simulink model "EL5101"  (Simulink 9.2)
settings: Solver=FixedStepDiscrete  StartTime=0.0  StopTime=inf  FixedStep=param.t_sample  RelTol=1e-3
undefined symbols (not defined in the file or in its folder): Angle_deg
libraries: simulink_extras x1, etherlab_lib x1
settings Model: Creator=schappler  LastModifiedBy=pkr_devpc  SimulationMode=external  ExtModeTrigDuration=10000  ExtModeArchiveMode=auto  ExtModeArchiveFileName=measurement_data  ExtModeArchiveDirName=/home/pkr_devpc/Schreibtisch/Git/3rrr_pkm/Versuchsstand/result  ExtModeLogAll=off
settings SolverCC: MinimalZcImpactIntegration=on
settings DataIOCC: LimitDataPoints=off  SaveFormat=Dataset  SignalLoggingSaveFormat=Dataset  SaveOutput=off  SignalLogging=off  SaveTime=off
settings OptimizationCC: BufferReuse=off  GlobalBufferReuse=off  ExpressionFolding=off  LocalBlockOutputs=off  LifeSpan=auto  OptimizeDataStoreBuffers=off  BusAssignmentInplaceUpdate=off
settings DebuggingCC: ReadBeforeWriteMsg=DisableAll  WriteAfterWriteMsg=DisableAll  WriteAfterReadMsg=DisableAll  UnderspecifiedInitializationDetection=Simplified  MergeDetectMultiDrivingBlocksExec=error  MultiTaskDSMMsg=none  FcnCallInpInsideContextMsg=error  StateNameClashWarn=none  SFUnexpectedBacktrackingDiag=error  SFNoUnconditionalDefaultTransitionDiag=error  SFExecutionAtInitializationDiag=warning
settings HardwareCC: ProdBitPerPointer=64  ProdBitPerSizeT=64  ProdBitPerPtrDiffT=64  ProdLargestAtomicFloat=Float  ProdIntDivRoundTo=Zero  ProdEndianess=LittleEndian  ProdWordSize=64  ProdHWDeviceType=Intel->x86-64 (Windows64)
settings ModelReferenceCC: UpdateModelReferenceTargets=IfOutOfDate  PropagateSignalLabelsOutOfModel=on
settings SFSimCC: SFSimEcho=off  SimUseLocalCustomCode=on
settings RTWCC: SystemTargetFile=etherlab.tlc  TemplateMakefile=etherlab_hrt.tmf  Description=EtherLab PREEMT_RT Real-Time Target  GenerateReport=on  RTWUseLocalCustomCode=on  LaunchReport=on
settings CodeAppCC: StateflowObjectComments=off
settings STFCustomTargetCC: TargetLangStandard=C99 (ISO)  SystemTargetFile=etherlab.tlc
settings GRTTargetCC: TargetLangStandard=C99 (ISO)  ParMdlRefBuildCompliant=off  CompOptLevelCompliant=off  ConcurrentExecutionCompliant=off  GeneratePreprocessorConditionals=Use local settings  MatFileLogging=off  CPPClassGenCompliant=off  UseToolchainInfoCompliant=off  ExtMode=on  ExtModeStaticAlloc=on  ExtModeStaticAllocSize=2000000000  ExtModeMexArgs='10.144.130.139' 0 17725  RTWCAPISignals=on  RTWCAPIParams=on
settings CustomProperty: DataType=int32  Value=2
settings ConfigComp: CovMetricSettings=dwe  CovHtmlReporting=off  CovSaveCumulativeToWorkspaceVar=off  CovSaveSingleToWorkspaceVar=off  CovExternalEMLEnable=on

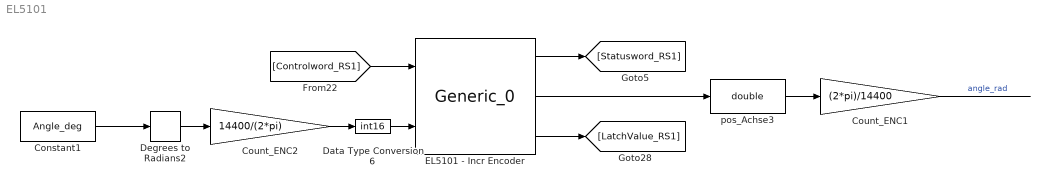
== system EL5101 ==
  Constant1 : Constant  Value=Angle_deg  SampleTime=-1
  Count_ENC1 : Gain  Gain=(2*pi)/14400  ParamDataTypeStr=double  OutDataTypeStr=double
  Count_ENC2 : Gain  Gain=14400/(2*pi)  ParamDataTypeStr=double  OutDataTypeStr=double
  Data Type Conversion6 : DataTypeConversion  OutDataTypeStr=int16
  Degrees to Radians2 : simulink_extras/Transformations/Degrees to Radians
  EL5101 - Incr Encoder : etherlab_lib/EtherCAT/Generic_0  master=0  index=8  rv=EL5101  param=[]  tsample=0.001  debug=0
  pos_Achse3 : DataTypeConversion  OutDataTypeStr=double
  wires:
  [Controlword_RS1] -> EL5101 - Incr Encoder/1
  Degrees to Radians2/1 -> Count_ENC2/1
  EL5101 - Incr Encoder/3 -> [LatchValue_RS1]
  Data Type Conversion6/1 -> EL5101 - Incr Encoder/2
  Count_ENC2/1 -> Data Type Conversion6/1
  EL5101 - Incr Encoder/1 -> [Statusword_RS1]
  EL5101 - Incr Encoder/2 -> pos_Achse3/1
  Constant1/1 -> Degrees to Radians2/1
  pos_Achse3/1 -> Count_ENC1/1
  Count_ENC1/1 -> ?  "angle_rad"
